simulink library "visualization_lib"  (R2016b)
settings: Solver=VariableStepAuto  StartTime=0.0  StopTime=10.0  RelTol=1e-3
libraries: ground_visualization_lib x1, gs_prediction_lib x1, rotation_visualization_lib x1, sun_vector_lib x1, time_coord_rotation_lib x1
settings Model: Creator=Sean  LastModifiedBy=Sean

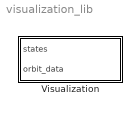
== system visualization_lib ==
  Visualization : Subsystem

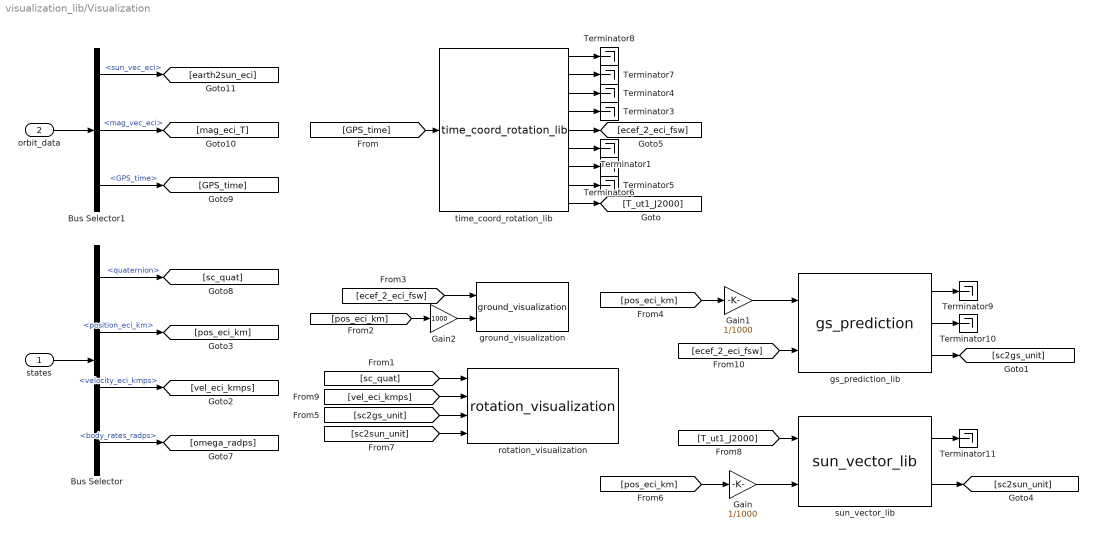
== system visualization_lib/Visualization ==
  states : Inport  OutDataTypeStr=Bus: states
  orbit_data : Inport  Port=2  OutDataTypeStr=Bus: orbit_data
  Bus Selector : BusSelector  OutputSignals=quaternion,position_eci_km,velocity_eci_kmps,body_rates_radps
  Bus Selector1 : BusSelector  OutputSignals=sun_vec_eci,mag_vec_eci,GPS_time
  Gain : Gain  Gain=1/1000
  Gain1 : Gain  Gain=1/1000
  Gain2 : Gain  Gain=1000
  Terminator{1,3..11} (10 alike) : Terminator
  ground_visualization : ground_visualization_lib/ground_visualization
  gs_prediction_lib : gs_prediction_lib/gs_prediction
  rotation_visualization : rotation_visualization_lib/rotation_visualization
  sun_vector_lib : sun_vector_lib/sun_vector_lib
  time_coord_rotation_lib : time_coord_rotation_lib/time_coord_rotation_lib
  wires:
  [pos_eci_km] -> Gain2/1
  Gain2/1 -> ground_visualization/2
  [vel_eci_kmps] -> rotation_visualization/2
  time_coord_rotation_lib/2 -> Terminator7/1
  time_coord_rotation_lib/3 -> Terminator4/1
  time_coord_rotation_lib/4 -> Terminator3/1
  time_coord_rotation_lib/5 -> [ecef_2_eci_fsw]
  time_coord_rotation_lib/6 -> Terminator1/1
  time_coord_rotation_lib/7 -> Terminator6/1
  time_coord_rotation_lib/8 -> Terminator5/1
  time_coord_rotation_lib/9 -> [T_ut1_J2000]
  [GPS_time] -> time_coord_rotation_lib/1
  time_coord_rotation_lib/1 -> Terminator8/1
  Bus Selector1/1 -> [earth2sun_eci]  "<sun_vec_eci>"
  Bus Selector1/2 -> [mag_eci_T]  "<mag_vec_eci>"
  Bus Selector1/3 -> [GPS_time]  "<GPS_time>"
  Bus Selector/1 -> [sc_quat]  "<quaternion>"
  Bus Selector/4 -> [omega_radps]  "<body_rates_radps>"
  Bus Selector/2 -> [pos_eci_km]  "<position_eci_km>"
  Bus Selector/3 -> [vel_eci_kmps]  "<velocity_eci_kmps>"
  orbit_data/1 -> Bus Selector1/1
  states/1 -> Bus Selector/1
  [sc_quat] -> rotation_visualization/1
  [ecef_2_eci_fsw] -> ground_visualization/1
  [pos_eci_km] -> Gain1/1
  [ecef_2_eci_fsw] -> gs_prediction_lib/2
  gs_prediction_lib/2 -> Terminator10/1
  gs_prediction_lib/3 -> [sc2gs_unit]
  gs_prediction_lib/1 -> Terminator9/1
  [pos_eci_km] -> Gain/1
  sun_vector_lib/1 -> Terminator11/1
  [T_ut1_J2000] -> sun_vector_lib/1
  sun_vector_lib/2 -> [sc2sun_unit]
  Gain/1 -> sun_vector_lib/2
  Gain1/1 -> gs_prediction_lib/1
  [sc2gs_unit] -> rotation_visualization/3
  [sc2sun_unit] -> rotation_visualization/4
